simulink model "Simulacion_punto_6"  (R2020a)
settings: Solver=VariableStepAuto  StartTime=0.0  StopTime=25.0  RelTol=1e-3
settings Model: Creator=Marco  LastModifiedBy=Marco

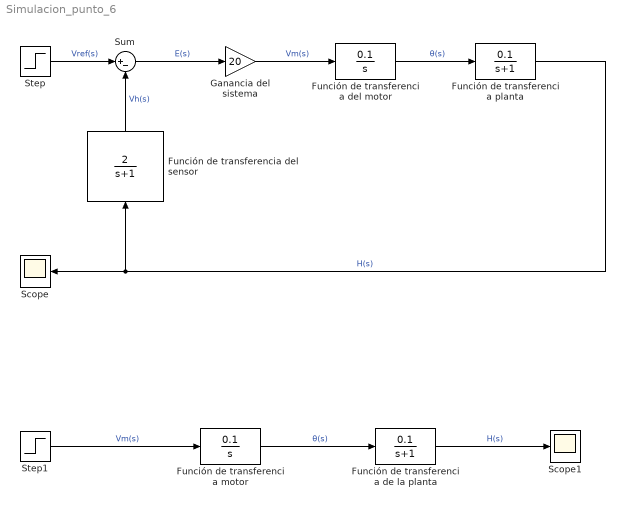
== system Simulacion_punto_6 ==
  " Función de transferencia del motor" : TransferFcn  Numerator=[0.1]  Denominator=[1 0]
  " Función de transferencia motor" : TransferFcn  Numerator=[0.1]  Denominator=[1 0]
  Función de transferencia de la planta : TransferFcn  Numerator=[0.1]  Denominator=[1 1]
  "Función de transferencia del sensor          " : TransferFcn  Numerator=[2]  Denominator=[1 1]
  Función de transferencia planta : TransferFcn  Numerator=[0.1]  Denominator=[1 1]
  Ganancia del sistema : Gain  Gain=20
  Scope : Scope
  Scope1 : Scope
  Step : Step  SampleTime=0
  Step1 : Step  SampleTime=0
  Sum : Sum  Inputs=|+-
  wires:
  " Función de transferencia del motor"/1 -> Función de transferencia planta/1  "θ(s)"
  Función de transferencia planta/1 -> "Función de transferencia del sensor          "/1, Scope/1  "H(s)"
  Step/1 -> Sum/1  "Vref(s)"
  Sum/1 -> Ganancia del sistema/1  "E(s)"
  "Función de transferencia del sensor          "/1 -> Sum/2  "Vh(s)"
  Ganancia del sistema/1 -> " Función de transferencia del motor"/1  "Vm(s)"
  Step1/1 -> " Función de transferencia motor"/1  "Vm(s)"
  Función de transferencia de la planta/1 -> Scope1/1  "H(s)"
  " Función de transferencia motor"/1 -> Función de transferencia de la planta/1  "θ(s)"
